simulink model "PFC_SIL_model"  (R2021a)
settings: Solver=VariableStepAuto  StartTime=0.0  StopTime=1  MaxStep=1e-5  RelTol=1e-3
values from neighbouring files (symbols this model uses):
  ki_current = 140/3    (= 46.6666666667)    [PFC_drscrete.m]
  ki_volt = 0.4    [PFC_drscrete.m]
  kp_curr = 0.027    [PFC_drscrete.m]
  kp_volt = 0.03    [PFC_drscrete.m]
  Po = 15000/3    (= 5000)    [PFC_drscrete.m]
  Ramp = 0.008    [PFC_drscrete.m]
  ramp_initial = 0.2    [PFC_drscrete.m]
  ramp_sat_max = 0.95    [PFC_drscrete.m]
  ramp_sat_min = 0.2    [PFC_drscrete.m]
  Ro = 100e3    (= 100000)    [PFC_drscrete.m]
  Softstart_th = 30    [PFC_drscrete.m]
  Vm = 400    [PFC_drscrete.m]
  Vo = 100    [PFC_drscrete.m]
undefined symbols (not defined in the file or in its folder): DiscIntNeverNeededParam, T_Finished, T_step
libraries: spsSeriesRLCBranchLib x34, simulink x19, spsMosfetLib x8, spsPWMGeneratorDCDCLib x8, spsControlledVoltageSourceLib x6, spsGroundLib x6, spsVoltageMeasurementLib x6, spsCurrentMeasurementLib x3, pid_lib x2, spsDiodeLib x2, spspowerguiLib x1
(part 1 of 2)
settings Model: Creator=houma  LastModifiedBy=prizm
settings SolverCC: AlgebraicLoopSolver=TrustRegion
settings DataIOCC: ReturnWorkspaceOutputs=off
settings DebuggingCC: SFMachineParentedDataDiag=warning  ArithmeticOperatorsInVariantConditions=warning
settings SFSimCC: SimUseLocalCustomCode=off  CustomCodeUndefinedFunction=UseInterfaceOnly
settings RTWCC: RTWUseLocalCustomCode=off

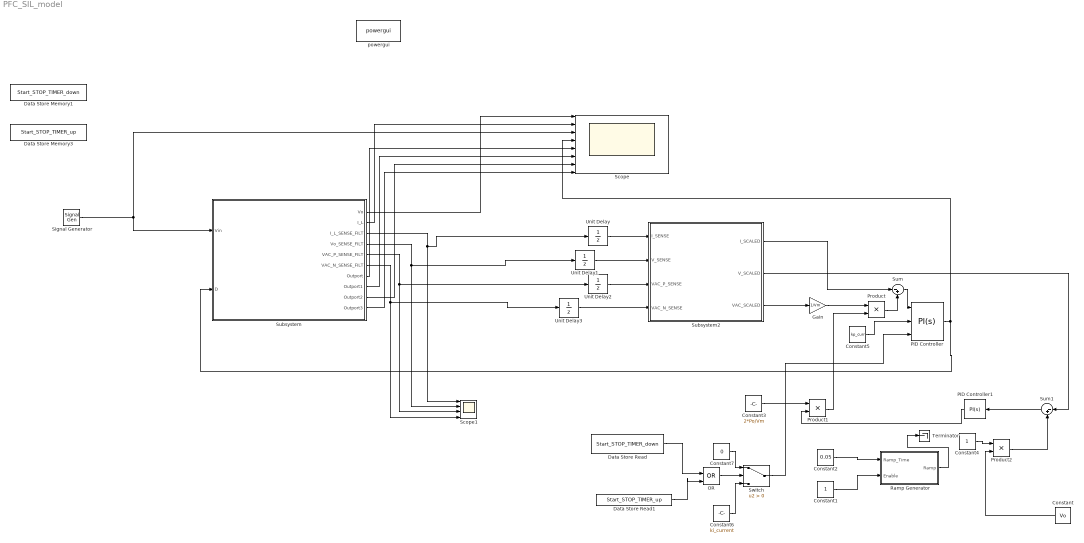
== system PFC_SIL_model ==
  Constant : Constant  Value=Vo
  Constant1 : Constant
  Constant2 : Constant  Value=0.05
  Constant3 : Constant  Value=2*Po/Vm
  Constant4 : Constant
  Constant5 : Constant  Value=kp_curr
  Constant6 : Constant  Value=ki_current
  Constant7 : Constant  Value=0
  Data Store Memory1 : DataStoreMemory  DataStoreName=Start_STOP_TIMER_down  ReadBeforeWriteMsg=warning  WriteAfterWriteMsg=warning  WriteAfterReadMsg=warning  ShowAdditionalParam=off
  Data Store Memory3 : DataStoreMemory  DataStoreName=Start_STOP_TIMER_up  ReadBeforeWriteMsg=warning  WriteAfterWriteMsg=warning  WriteAfterReadMsg=warning  ShowAdditionalParam=off
  Data Store Read : DataStoreRead  DataStoreName=Start_STOP_TIMER_down  IndexOptions=Index vector (dialog)  Indices=1  OutputSizes=1
  Data Store Read1 : DataStoreRead  DataStoreName=Start_STOP_TIMER_up  IndexOptions=Index vector (dialog)  Indices=1  OutputSizes=1
  Gain : Gain  Gain=1/Vm
  OR : Logic  Operator=OR  IconShape=distinctive  AllPortsSameDT=off  OutDataTypeStr=boolean
  PID Controller : pid_lib/PID Controller  Controller=PI  Form=Parallel  TimeDomain=Continuous-time  UseExternalTs=off  SampleTime=-1  IntegratorMethod=Forward Euler  FilterMethod=Forward Euler  ControllerParametersSource=external  P=0.027  I=140*2  D=0.0002  UseFilter=on  N=100  TunerSelectOption=Transfer Function Based (PID Tuner App)  InitialConditionSource=internal  InitialConditionForIntegrator=0  InitialConditionForFilter=0  DifferentiatorICPrevScaledInput=0  ExternalReset=none  TrackingMode=off  Kt=1  LimitOutput=on  SatLimitsSource=internal  UpperSaturationLimit=0.95  LowerSaturationLimit=0.05  LinearizeAsGain=off  AntiWindupMode=none  Kb=1  POutMin=[]  POutMax=[]  IOutMin=[]  IOutMax=[]  DOutMin=[]  DOutMax=[]  NOutMin=[]  NOutMax=[]  SumOutMin=[]  SumOutMax=[]  SaturationOutMin=[]  SaturationOutMax=[]  PParamMin=[]  PParamMax=[]  IParamMin=[]  IParamMax=[]  DParamMin=[]  DParamMax=[]  NParamMin=[]  NParamMax=[]  KbParamMin=[]  KbParamMax=[]  KtParamMin=[]  KtParamMax=[]  KbOutMin=[]  KbOutMax=[]  KtOutMin=[]  KtOutMax=[]  IntegratorOutMin=[]  IntegratorOutMax=[]  FilterOutMin=[]  FilterOutMax=[]  SumI1OutMin=[]  SumI1OutMax=[]  SumI2OutMin=[]  SumI2OutMax=[]  SumI3OutMin=[]  SumI3OutMax=[]  SumI4OutMin=[]  SumI4OutMax=[]  SumDOutMin=[]  SumDOutMax=[]  DifferentiatorOutMin=[]  DifferentiatorOutMax=[]  FilterDiffOutCoefMin=[]  FilterDiffOutCoefMax=[]  ReciprocalOutMin=[]  ReciprocalOutMax=[]  SumDenOutMin=[]  SumDenOutMax=[]  SumNumOutMin=[]  SumNumOutMax=[]  DivideOutMin=[]  DivideOutMax=[]  UdiffTsProdOutMin=[]  UdiffTsProdOutMax=[]  NTsProdOutMin=[]  NTsProdOutMax=[]  UintegralTsProdOutMin=[]  UintegralTsProdOutMax=[]  UngainTsProdOutMin=[]  UngainTsProdOutMax=[]  IntegratorContinuousStateAttributes=''  IntegratorStateMustResolveToSignalObject=off  IntegratorRTWStateStorageClass=Auto  FilterContinuousStateAttributes=''  FilterStateMustResolveToSignalObject=off  FilterRTWStateStorageClass=Auto  ParallelPVariant=ExternalParameters  IdealPVariant=Disabled  IVariant=ExternalParameters  DVariant=Disabled  IntegratorVariant=Continuous  SatVariant=Enabled  AWVariant=Passthrough  PCopyVariant=Disabled  TRVariant=Disabled  FdbkBlocksVariant=Forward  IdealPFdbkVariant=Disabled  SatFdbkVariant=Disabled  DerivativeFilterVariant=Disabled  NVariant=Disabled  NCopyVariant=Disabled_SignalSpec  FilterICVariant=Disabled  IntegratorICVariant=InternalICs  ExternalResetVariant=Disabled  TRSumVariant=Passthrough  SumFdbkVariant=Disabled  SumVariant=Sum_PI  TsampFilterVariant=InternalTs  TsampNgainVariant=Passthrough  TsampIntegralVariant=Passthrough  ExternalSaturationOutDataTypeStr=Inherit: Same as second input
  PID Controller1 : pid_lib/PID Controller  Controller=PI  Form=Parallel  TimeDomain=Continuous-time  UseExternalTs=off  SampleTime=-1  IntegratorMethod=Forward Euler  FilterMethod=Forward Euler  ControllerParametersSource=internal  P=kp_volt  I=ki_volt  D=0  UseFilter=on  N=100  TunerSelectOption=Transfer Function Based (PID Tuner App)  InitialConditionSource=internal  InitialConditionForIntegrator=0  InitialConditionForFilter=0  DifferentiatorICPrevScaledInput=0  ExternalReset=none  TrackingMode=off  Kt=1  LimitOutput=on  SatLimitsSource=internal  UpperSaturationLimit=1  LowerSaturationLimit=0  LinearizeAsGain=off  AntiWindupMode=none  Kb=1  POutMin=[]  POutMax=[]  IOutMin=[]  IOutMax=[]  DOutMin=[]  DOutMax=[]  NOutMin=[]  NOutMax=[]  SumOutMin=[]  SumOutMax=[]  SaturationOutMin=[]  SaturationOutMax=[]  PParamMin=[]  PParamMax=[]  IParamMin=[]  IParamMax=[]  DParamMin=[]  DParamMax=[]  NParamMin=[]  NParamMax=[]  KbParamMin=[]  KbParamMax=[]  KtParamMin=[]  KtParamMax=[]  KbOutMin=[]  KbOutMax=[]  KtOutMin=[]  KtOutMax=[]  IntegratorOutMin=[]  IntegratorOutMax=[]  FilterOutMin=[]  FilterOutMax=[]  SumI1OutMin=[]  SumI1OutMax=[]  SumI2OutMin=[]  SumI2OutMax=[]  SumI3OutMin=[]  SumI3OutMax=[]  SumI4OutMin=[]  SumI4OutMax=[]  SumDOutMin=[]  SumDOutMax=[]  DifferentiatorOutMin=[]  DifferentiatorOutMax=[]  FilterDiffOutCoefMin=[]  FilterDiffOutCoefMax=[]  ReciprocalOutMin=[]  ReciprocalOutMax=[]  SumDenOutMin=[]  SumDenOutMax=[]  SumNumOutMin=[]  SumNumOutMax=[]  DivideOutMin=[]  DivideOutMax=[]  UdiffTsProdOutMin=[]  UdiffTsProdOutMax=[]  NTsProdOutMin=[]  NTsProdOutMax=[]  UintegralTsProdOutMin=[]  UintegralTsProdOutMax=[]  UngainTsProdOutMin=[]  UngainTsProdOutMax=[]  IntegratorContinuousStateAttributes=''  IntegratorStateMustResolveToSignalObject=off  IntegratorRTWStateStorageClass=Auto  FilterContinuousStateAttributes=''  FilterStateMustResolveToSignalObject=off  FilterRTWStateStorageClass=Auto  ParallelPVariant=InternalParameters  IdealPVariant=Disabled  IVariant=InternalParameters  DVariant=Disabled  IntegratorVariant=Continuous  SatVariant=Enabled  AWVariant=Passthrough  PCopyVariant=Disabled  TRVariant=Disabled  FdbkBlocksVariant=Forward  IdealPFdbkVariant=Disabled  SatFdbkVariant=Disabled  DerivativeFilterVariant=Disabled  NVariant=Disabled  NCopyVariant=Disabled_SignalSpec  FilterICVariant=Disabled  IntegratorICVariant=InternalICs  ExternalResetVariant=Disabled  TRSumVariant=Passthrough  SumFdbkVariant=Disabled  SumVariant=Sum_PI  TsampFilterVariant=InternalTs  TsampNgainVariant=Passthrough  TsampIntegralVariant=Passthrough  ExternalSaturationOutDataTypeStr=Inherit: Same as second input
  Product : Product
  Product1 : Product
  Product2 : Product
  Ramp Generator : Subsystem
  Scope : Scope  NumInputPorts=8
  Scope1 : Scope  NumInputPorts=4
  Signal Generator : SignalGenerator  Amplitude=Vm  Frequency=60
  Subsystem : Subsystem
  Subsystem2 : Subsystem
  Sum : Sum  Inputs=|-+
  Sum1 : Sum  Inputs=|-+
  Switch : Switch  Criteria=u2 > Threshold
  Terminator : Terminator
  Unit Delay{,1..3} (4 alike) : UnitDelay  SampleTime=-1  HasFrameUpgradeWarning=on
  powergui : spspowerguiLib/powergui  Priority=1  SimulationMode=Continuous  SampleTime=50e-6  frequency=60  Iterations=50  frequencyindice=0  Pbase=100e6  ErrMax=1e-4  UnitsV=kV  UnitsW=MW  buscounter=0  FunctionMessages=off  echomessages=off  EnableUseOfTLC=off  CurrentSourceSwitches=off  DisableSnubberDevices=off  DisableRonSwitches=off  DisableVfSwitches=off  DisplayEquations=off  AutomaticDiscreteSolvers=off  SolverType=Tustin/Backward Euler (TBE)  Interpol=off  ExternalGateDelay=off  methode=off  Ts=100  x0status=blocks  SPID=on  SwTol=0  HookPort=off  NonlinearTolerance=1e-4  nMaxIteration=100  ContinueOnMaxIteration=off  RestoreLinks=warning  ResistiveCurrentMeasurement=off  Frange=[0:2:500]  Ylog=off  Xlog=on  ShowGrid=off  save=off  variable=ZData  structure=0  ZoomFFT=off  StartTime=0.0  cycles=1  DisplayStyle=1  fundamental=60  FreqAxis=off  MaxFrequency=1000  frequencyindicesteady=1  RmsSteady=1  display=off
  wires:
  Subsystem2/1(I_SCALED) -> Sum/1
  Subsystem/3(I_L_SENSE_FILT) -> Scope1/1, Unit Delay/1
  Gain/1 -> Product/1
  Product/1 -> Sum/2
  Subsystem/6(VAC_N_SENSE_FILT) -> Scope1/4, Unit Delay3/1
  Subsystem/4(Vo_SENSE_FILT) -> Scope1/2, Unit Delay1/1
  Subsystem2/3(VAC_SCALED) -> Gain/1
  Unit Delay/1 -> Subsystem2/1(I_SENSE)
  Unit Delay1/1 -> Subsystem2/2(V_SENSE)
  Unit Delay2/1 -> Subsystem2/3(VAC_P_SENSE)
  Subsystem/1(Vo) -> Scope/1
  Subsystem/5(VAC_P_SENSE_FILT) -> Scope1/3, Unit Delay2/1
  Unit Delay3/1 -> Subsystem2/4(VAC_N_SENSE)
  Subsystem/2(I_L) -> Scope/2
  Sum/1 -> PID Controller/1
  Signal Generator/1 -> Scope/3, Subsystem/1(Vin)
  PID Controller/1 -> Scope/4, Subsystem/2(D)
  Constant3/1 -> Product1/1
  Product1/1 -> Product/2
  Subsystem2/2(V_SCALED) -> Sum1/1
  Sum1/1 -> PID Controller1/1
  PID Controller1/1 -> Product1/2
  Constant/1 -> Product2/2
  Subsystem/7(Outport) -> Scope/5
  Subsystem/8(Outport1) -> Scope/6
  Subsystem/9(Outport2) -> Scope/7
  Subsystem/10(Outport3) -> Scope/8
  Ramp Generator/1(Ramp) -> Terminator/1
  Product2/1 -> Sum1/2
  Constant1/1 -> Ramp Generator/2(Enable)
  Constant2/1 -> Ramp Generator/1(Ramp_Time)
  Constant4/1 -> Product2/1
  Constant5/1 -> PID Controller/2
  Switch/1 -> PID Controller/3
  Data Store Read/1 -> OR/1
  Data Store Read1/1 -> OR/2
  OR/1 -> Switch/2
  Constant7/1 -> Switch/1
  Constant6/1 -> Switch/3

== system PFC_SIL_model/Ramp Generator ==
  Ramp_Time : Inport
  Enable : Inport  Port=2
  Divide : Product  Inputs=*/  RndMeth=Simplest  OutDataTypeStr=Inherit: Same as first input
  NOT : Logic  Operator=NOT  IconShape=distinctive  AllPortsSameDT=off  OutDataTypeStr=boolean
  One : Constant  SampleTime=-1
  Ramp Generator : DiscreteIntegrator  IntegratorMethod=Accumulation: Forward Euler  gainval=1  ExternalReset=sampled level  SampleTime=-1  RndMeth=Simplest  LimitOutput=on  UpperSaturationLimit=1  LowerSaturationLimit=0  ICPrevOutput=DiscIntNeverNeededParam  ICPrevScaledInput=DiscIntNeverNeededParam
  Sample_Time : Gain  Gain=0.00001  RndMeth=Simplest  OutDataTypeStr=Inherit: Same as input
  Ramp : Outport
  wires:
  Divide/1 -> Sample_Time/1
  Ramp Generator/1 -> Ramp/1  "Eps"
  Sample_Time/1 -> Ramp Generator/1
  One/1 -> Divide/1
  Ramp_Time/1 -> Divide/2
  Enable/1 -> NOT/1
  NOT/1 -> Ramp Generator/2

== system PFC_SIL_model/Subsystem ==
  Vin : Inport
  D : Inport  Port=2
  Subsystem3 : Subsystem
  Subsystem4 : Subsystem
  Subsystem5 : Subsystem
  Vo : Outport  VectorParamsAs1DForOutWhenUnconnected=off
  I_L : Outport  Port=2  VectorParamsAs1DForOutWhenUnconnected=off
  I_L_SENSE_FILT : Outport  Port=3  VectorParamsAs1DForOutWhenUnconnected=off
  Vo_SENSE_FILT : Outport  Port=4  VectorParamsAs1DForOutWhenUnconnected=off
  VAC_P_SENSE_FILT : Outport  Port=5  VectorParamsAs1DForOutWhenUnconnected=off
  VAC_N_SENSE_FILT : Outport  Port=6  VectorParamsAs1DForOutWhenUnconnected=off
  Outport : Outport  Port=7
  Outport1 : Outport  Port=8
  Outport2 : Outport  Port=9
  Outport3 : Outport  Port=10
  wires:
  Subsystem3/1(VAC_N_Sense_FILT) -> VAC_N_SENSE_FILT/1  "VAC_N_SENSE_FILT"
  Subsystem5/3(I_L_Sense_FILT) -> I_L_SENSE_FILT/1  "I_L_SENSE_FILT"
  Subsystem5/1(Vo) -> Vo/1  "Vo"
  Vin/1 -> Subsystem3/1(VAC_IN), Subsystem4/1(VAC_IN), Subsystem5/1(Vin)
  Subsystem5/4(Vo_Sense_FILT) -> Vo_SENSE_FILT/1  "Vo_SENSE_FILT"
  D/1 -> Subsystem5/2(D)
  Subsystem4/1(VAC_P_Sense_FILT) -> VAC_P_SENSE_FILT/1  "VAC_P_SENSE_FILT"
  Subsystem5/2(I_L) -> I_L/1
  Subsystem5/5(Outport) -> Outport/1
  Subsystem5/6(Outport1) -> Outport1/1
  Subsystem5/7(Outport2) -> Outport2/1
  Subsystem5/8(Outport3) -> Outport3/1

== system PFC_SIL_model/Subsystem2 ==
  I_SENSE : Inport
  V_SENSE : Inport  Port=2
  VAC_P_SENSE : Inport  Port=3
  VAC_N_SENSE : Inport  Port=4
  Gain : Gain  Gain=307.39
  Gain1 : Gain  Gain=230.79
  Gain2 : Gain  Gain=230.79
  Subsystem1 : Subsystem  mask{Gain=0.025, Vref=2.5}
      mask prompts: Gain "Gain (mV/A)"; Vref "reference Voltage"
  Sum : Sum  Inputs=|+-
  I_SCALED : Outport  VectorParamsAs1DForOutWhenUnconnected=off
  V_SCALED : Outport  Port=2  VectorParamsAs1DForOutWhenUnconnected=off
  VAC_SCALED : Outport  Port=3  VectorParamsAs1DForOutWhenUnconnected=off
  wires:
  Sum/1 -> VAC_SCALED/1  "VAC_SCALED"
  V_SENSE/1 -> Gain/1
  Subsystem1/1(I_Scaled) -> I_SCALED/1  "I_SCALED"
  Gain/1 -> V_SCALED/1  "V_SCALED"
  VAC_N_SENSE/1 -> Gain2/1
  Gain1/1 -> Sum/1
  Gain2/1 -> Sum/2
  I_SENSE/1 -> Subsystem1/1(I_ADC)
  VAC_P_SENSE/1 -> Gain1/1

== system PFC_SIL_model/Subsystem/Subsystem3 ==
  VAC_IN : Inport
  Controlled Voltage Source3 : spsControlledVoltageSourceLib/Controlled Voltage Source  Initialize=on  Source_Type=AC  Amplitude=0  Phase=0  Frequency=0  Measurements=None
  Diode1 : spsDiodeLib/Diode  Ron=0.001  Lon=0  Vf=0.8  IC=0  UseSnubber=0  Rs=1e9  Cs=0  Measurements=off
  Ground3 : spsGroundLib/Ground  LConnTagsString=a
  Series RLC Branch21 : spsSeriesRLCBranchLib/Series RLC Branch  LConnTagsString=__new0  RConnTagsString=__new0  BranchType=R  Resistance=15000  Inductance=1e-3  SetiL0=off  InitialCurrent=0  Capacitance=1e-6  Setx0=off  InitialVoltage=0  Measurements=None
  Series RLC Branch22 : spsSeriesRLCBranchLib/Series RLC Branch  LConnTagsString=__new0  RConnTagsString=__new0  BranchType=C  Resistance=4700  Inductance=1e-3  SetiL0=off  InitialCurrent=0  Capacitance=1e-9  Setx0=off  InitialVoltage=0  Measurements=None
  Series RLC Branch23 : spsSeriesRLCBranchLib/Series RLC Branch  LConnTagsString=__new0  RConnTagsString=__new0  BranchType=R  Resistance=15000  Inductance=1e-3  SetiL0=off  InitialCurrent=0  Capacitance=1e-6  Setx0=off  InitialVoltage=0  Measurements=None
  Series RLC Branch24 : spsSeriesRLCBranchLib/Series RLC Branch  LConnTagsString=__new0  RConnTagsString=__new0  BranchType=C  Resistance=4700  Inductance=1e-3  SetiL0=off  InitialCurrent=0  Capacitance=1e-9  Setx0=off  InitialVoltage=0  Measurements=None
  Series RLC Branch25 : spsSeriesRLCBranchLib/Series RLC Branch  LConnTagsString=__new0  RConnTagsString=__new0  BranchType=R  Resistance=1.08e6  Inductance=1e-3  SetiL0=off  InitialCurrent=0  Capacitance=1e-6  Setx0=off  InitialVoltage=0  Measurements=None
  Series RLC Branch26 : spsSeriesRLCBranchLib/Series RLC Branch  LConnTagsString=__new0  RConnTagsString=__new0  BranchType=R  Resistance=4700  Inductance=1e-3  SetiL0=off  InitialCurrent=0  Capacitance=1e-6  Setx0=off  InitialVoltage=0  Measurements=None
  Series RLC Branch27 : spsSeriesRLCBranchLib/Series RLC Branch  LConnTagsString=__new0  RConnTagsString=__new0  BranchType=C  Resistance=4700  Inductance=1e-3  SetiL0=off  InitialCurrent=0  Capacitance=470e-12  Setx0=off  InitialVoltage=0  Measurements=None
  Voltage Measurement3 : spsVoltageMeasurementLib/Voltage Measurement  PhasorSimulation=off  OutputType=Complex  PSBequivalent=0
  VAC_N_Sense_FILT : Outport  VectorParamsAs1DForOutWhenUnconnected=off
  wires:
  VAC_IN/1 -> Controlled Voltage Source3/1
  Voltage Measurement3/1 -> VAC_N_Sense_FILT/1  "VAC_N_Sense_FILT"
  connections:
  Diode1/RConn1 -- Series RLC Branch25/LConn1
  Series RLC Branch26/RConn1 -- Series RLC Branch27/RConn1 -- Series RLC Branch22/RConn1 -- Series RLC Branch24/RConn1 -- Voltage Measurement3/LConn2 -- Ground3/LConn1 -- Controlled Voltage Source3/RConn1
  Controlled Voltage Source3/LConn1 -- Diode1/LConn1
  Series RLC Branch23/RConn1 -- Voltage Measurement3/LConn1 -- Series RLC Branch24/LConn1
  Series RLC Branch25/RConn1 -- Series RLC Branch27/LConn1 -- Series RLC Branch21/LConn1 -- Series RLC Branch26/LConn1
  Series RLC Branch21/RConn1 -- Series RLC Branch22/LConn1 -- Series RLC Branch23/LConn1

== system PFC_SIL_model/Subsystem/Subsystem4 ==
  VAC_IN : Inport
  Controlled Voltage Source2 : spsControlledVoltageSourceLib/Controlled Voltage Source  Initialize=on  Source_Type=AC  Amplitude=0  Phase=0  Frequency=0  Measurements=None
  Current Measurement : spsCurrentMeasurementLib/Current Measurement  PhasorSimulation=off  OutputType=Complex  PSBequivalent=0
  Diode : spsDiodeLib/Diode  Ron=0.001  Lon=0  Vf=0.8  IC=0  UseSnubber=0  Rs=1e9  Cs=0  Measurements=off
  Ground2 : spsGroundLib/Ground  LConnTagsString=a
  Scope : Scope
  Series RLC Branch14 : spsSeriesRLCBranchLib/Series RLC Branch  LConnTagsString=__new0  RConnTagsString=__new0  BranchType=R  Resistance=15000  Inductance=1e-3  SetiL0=off  InitialCurrent=0  Capacitance=1e-6  Setx0=off  InitialVoltage=0  Measurements=None
  Series RLC Branch15 : spsSeriesRLCBranchLib/Series RLC Branch  LConnTagsString=__new0  RConnTagsString=__new0  BranchType=C  Resistance=4700  Inductance=1e-3  SetiL0=off  InitialCurrent=0  Capacitance=1e-9  Setx0=off  InitialVoltage=0  Measurements=None
  Series RLC Branch16 : spsSeriesRLCBranchLib/Series RLC Branch  LConnTagsString=__new0  RConnTagsString=__new0  BranchType=R  Resistance=15000  Inductance=1e-3  SetiL0=off  InitialCurrent=0  Capacitance=1e-6  Setx0=off  InitialVoltage=0  Measurements=None
  Series RLC Branch17 : spsSeriesRLCBranchLib/Series RLC Branch  LConnTagsString=__new0  RConnTagsString=__new0  BranchType=C  Resistance=4700  Inductance=1e-3  SetiL0=off  InitialCurrent=0  Capacitance=1e-9  Setx0=off  InitialVoltage=0  Measurements=None
  Series RLC Branch18 : spsSeriesRLCBranchLib/Series RLC Branch  LConnTagsString=__new0  RConnTagsString=__new0  BranchType=R  Resistance=1.08e6  Inductance=1e-3  SetiL0=off  InitialCurrent=0  Capacitance=1e-6  Setx0=off  InitialVoltage=0  Measurements=None
  Series RLC Branch19 : spsSeriesRLCBranchLib/Series RLC Branch  LConnTagsString=__new0  RConnTagsString=__new0  BranchType=R  Resistance=4700  Inductance=1e-3  SetiL0=off  InitialCurrent=0  Capacitance=1e-6  Setx0=off  InitialVoltage=0  Measurements=None
  Series RLC Branch20 : spsSeriesRLCBranchLib/Series RLC Branch  LConnTagsString=__new0  RConnTagsString=__new0  BranchType=C  Resistance=4700  Inductance=1e-3  SetiL0=off  InitialCurrent=0  Capacitance=470e-12  Setx0=off  InitialVoltage=0  Measurements=None
  Voltage Measurement2 : spsVoltageMeasurementLib/Voltage Measurement  PhasorSimulation=off  OutputType=Complex  PSBequivalent=0
  VAC_P_Sense_FILT : Outport  VectorParamsAs1DForOutWhenUnconnected=off
  wires:
  VAC_IN/1 -> Controlled Voltage Source2/1
  Voltage Measurement2/1 -> VAC_P_Sense_FILT/1  "VAC_P_Sense_FILT"
  Current Measurement/1 -> Scope/1
  connections:
  Current Measurement/LConn1 -- Series RLC Branch18/RConn1
  Series RLC Branch19/LConn1 -- Series RLC Branch20/LConn1 -- Series RLC Branch14/LConn1 -- Current Measurement/RConn1
  Series RLC Branch14/RConn1 -- Series RLC Branch15/LConn1 -- Series RLC Branch16/LConn1
  Series RLC Branch16/RConn1 -- Voltage Measurement2/LConn1 -- Series RLC Branch17/LConn1
  Ground2/LConn1 -- Series RLC Branch20/RConn1 -- Series RLC Branch15/RConn1 -- Series RLC Branch17/RConn1 -- Voltage Measurement2/LConn2 -- Series RLC Branch19/RConn1 -- Controlled Voltage Source2/LConn1
  Series RLC Branch18/LConn1 -- Diode/RConn1
  Diode/LConn1 -- Controlled Voltage Source2/RConn1

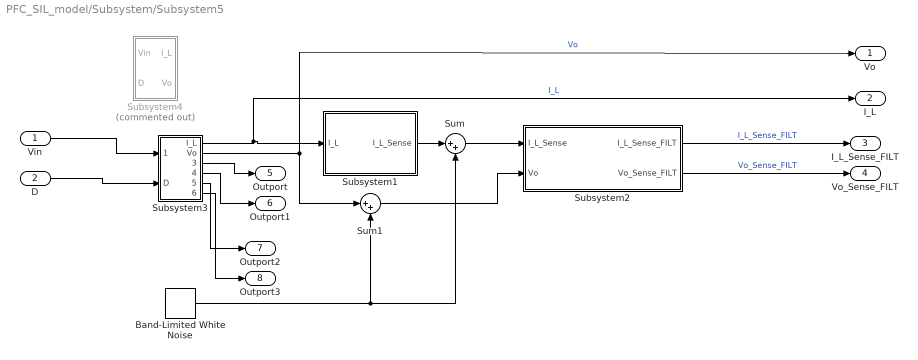
== system PFC_SIL_model/Subsystem/Subsystem5 ==
  Vin : Inport
  D : Inport  Port=2
  Band-Limited White Noise : simulink/Sources/Band-Limited White Noise  Cov=[0]  Ts=1/100e3  seed=[23341]
  Subsystem1 : Subsystem  mask{G_current=0.025, Vref=2.5}
      mask prompts: G_current "Current Gain (V/A)"; Vref "Reference Voltage"
  Subsystem2 : Subsystem
  Subsystem3 : Subsystem  mask{Lo=450e-6, Co=1.1e-3}
      mask prompts: Lo "PFC Inductance"; Co "Bus Capacitance"
  Subsystem4 : Subsystem  Commented=on  mask{Lo=450e-6, Co=1.1e-3}
      mask prompts: Lo "PFC Inductance"; Co "Bus Capacitance"
  Sum : Sum  Inputs=|++
  Sum1 : Sum  Inputs=|++
  Vo : Outport  VectorParamsAs1DForOutWhenUnconnected=off
  I_L : Outport  Port=2  VectorParamsAs1DForOutWhenUnconnected=off
  I_L_Sense_FILT : Outport  Port=3  VectorParamsAs1DForOutWhenUnconnected=off
  Vo_Sense_FILT : Outport  Port=4  VectorParamsAs1DForOutWhenUnconnected=off
  Outport : Outport  Port=5
  Outport1 : Outport  Port=6
  Outport2 : Outport  Port=7
  Outport3 : Outport  Port=8
  wires:
  D/1 -> Subsystem3/2(D)
  Subsystem2/2(Vo_Sense_FILT) -> Vo_Sense_FILT/1  "Vo_Sense_FILT"
  Subsystem2/1(I_L_Sense_FILT) -> I_L_Sense_FILT/1  "I_L_Sense_FILT"
  Vin/1 -> Subsystem3/1(Vin)
  Subsystem3/2(Vo) -> Sum1/1, Vo/1  "Vo"
  Subsystem3/1(I_L) -> I_L/1, Subsystem1/1(I_L)  "I_L"
  Band-Limited White Noise/1 -> Sum1/2, Sum/2
  Subsystem1/1(I_L_Sense) -> Sum/1
  Sum/1 -> Subsystem2/1(I_L_Sense)
  Sum1/1 -> Subsystem2/2(Vo)
  Subsystem3/3(Outport) -> Outport/1
  Subsystem3/4(Outport1) -> Outport1/1
  Subsystem3/5(Outport2) -> Outport2/1
  Subsystem3/6(Outport3) -> Outport3/1

== system PFC_SIL_model/Subsystem2/Subsystem1 ==
  I_ADC : Inport
  Constant3 : Constant  Value=Vref
  Gain : Gain  Gain=2
  Gain1 : Gain  Gain=1/Gain
  Sum : Sum  Inputs=|+-
  I_Scaled : Outport  VectorParamsAs1DForOutWhenUnconnected=off
  wires:
  Gain/1 -> Sum/1
  Constant3/1 -> Sum/2
  Gain1/1 -> I_Scaled/1  "I_Scaled"
  Sum/1 -> Gain1/1
  I_ADC/1 -> Gain/1

== system PFC_SIL_model/Subsystem/Subsystem5/Subsystem1 ==
  I_L : Inport
  Constant : Constant  Value=Vref
  Gain : Gain  Gain=G_current
  Sum : Sum  Inputs=|++
  I_L_Sense : Outport  VectorParamsAs1DForOutWhenUnconnected=off
  wires:
  Sum/1 -> I_L_Sense/1  "I_L_Sense"
  I_L/1 -> Gain/1
  Gain/1 -> Sum/1
  Constant/1 -> Sum/2

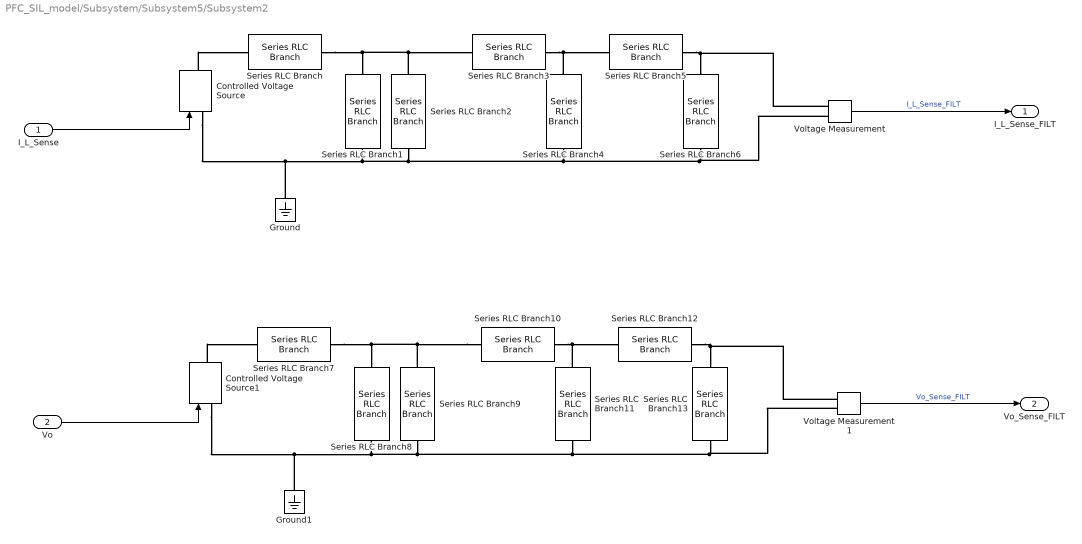
== system PFC_SIL_model/Subsystem/Subsystem5/Subsystem2 ==
  I_L_Sense : Inport
  Vo : Inport  Port=2
  Controlled Voltage Source : spsControlledVoltageSourceLib/Controlled Voltage Source  Initialize=on  Source_Type=AC  Amplitude=0  Phase=0  Frequency=0  Measurements=None
  Controlled Voltage Source1 : spsControlledVoltageSourceLib/Controlled Voltage Source  Initialize=on  Source_Type=AC  Amplitude=0  Phase=0  Frequency=0  Measurements=None
  Ground : spsGroundLib/Ground  LConnTagsString=a
  Ground1 : spsGroundLib/Ground  LConnTagsString=a
  Series RLC Branch{,1,3,5,8,10,12} (7 alike) : spsSeriesRLCBranchLib/Series RLC Branch  LConnTagsString=__new0  RConnTagsString=__new0  BranchType=R  Resistance=4700  Inductance=1e-3  SetiL0=off  InitialCurrent=0  Capacitance=1e-6  Setx0=off  InitialVoltage=0  Measurements=None
  Series RLC Branch{4,6,11,13} (4 alike) : spsSeriesRLCBranchLib/Series RLC Branch  LConnTagsString=__new0  RConnTagsString=__new0  BranchType=C  Resistance=4700  Inductance=1e-3  SetiL0=off  InitialCurrent=0  Capacitance=1e-9  Setx0=off  InitialVoltage=0  Measurements=None
  Series RLC Branch2 : spsSeriesRLCBranchLib/Series RLC Branch  LConnTagsString=__new0  RConnTagsString=__new0  BranchType=C  Resistance=4700  Inductance=1e-3  SetiL0=off  InitialCurrent=0  Capacitance=470e-12  Setx0=off  InitialVoltage=0  Measurements=None
  Series RLC Branch7 : spsSeriesRLCBranchLib/Series RLC Branch  LConnTagsString=__new0  RConnTagsString=__new0  BranchType=R  Resistance=1.44e6  Inductance=1e-3  SetiL0=off  InitialCurrent=0  Capacitance=1e-6  Setx0=off  InitialVoltage=0  Measurements=None
  Series RLC Branch9 : spsSeriesRLCBranchLib/Series RLC Branch  LConnTagsString=__new0  RConnTagsString=__new0  BranchType=C  Resistance=4700  Inductance=1e-3  SetiL0=off  InitialCurrent=0  Capacitance=470e-12  Setx0=off  InitialVoltage=0  Measurements=None
  Voltage Measurement : spsVoltageMeasurementLib/Voltage Measurement  PhasorSimulation=off  OutputType=Complex  PSBequivalent=0
  Voltage Measurement1 : spsVoltageMeasurementLib/Voltage Measurement  PhasorSimulation=off  OutputType=Complex  PSBequivalent=0
  I_L_Sense_FILT : Outport  VectorParamsAs1DForOutWhenUnconnected=off
  Vo_Sense_FILT : Outport  Port=2  VectorParamsAs1DForOutWhenUnconnected=off
  wires:
  I_L_Sense/1 -> Controlled Voltage Source/1
  Voltage Measurement/1 -> I_L_Sense_FILT/1  "I_L_Sense_FILT"
  Vo/1 -> Controlled Voltage Source1/1
  Voltage Measurement1/1 -> Vo_Sense_FILT/1  "Vo_Sense_FILT"
  connections:
  Series RLC Branch3/RConn1 -- Series RLC Branch4/LConn1 -- Series RLC Branch5/LConn1
  Series RLC Branch5/RConn1 -- Voltage Measurement/LConn1 -- Series RLC Branch6/LConn1
  Controlled Voltage Source/LConn1 -- Ground/LConn1 -- Voltage Measurement/LConn2 -- Series RLC Branch6/RConn1 -- Series RLC Branch4/RConn1 -- Series RLC Branch2/RConn1 -- Series RLC Branch1/RConn1
  Series RLC Branch/RConn1 -- Series RLC Branch2/LConn1 -- Series RLC Branch3/LConn1 -- Series RLC Branch1/LConn1
  Controlled Voltage Source/RConn1 -- Series RLC Branch/LConn1
  Voltage Measurement1/LConn2 -- Series RLC Branch13/RConn1 -- Series RLC Branch11/RConn1 -- Ground1/LConn1 -- Controlled Voltage Source1/LConn1 -- Series RLC Branch8/RConn1 -- Series RLC Branch9/RConn1
  Series RLC Branch10/LConn1 -- Series RLC Branch9/LConn1 -- Series RLC Branch8/LConn1 -- Series RLC Branch7/RConn1
  Series RLC Branch11/LConn1 -- Series RLC Branch12/LConn1 -- Series RLC Branch10/RConn1
  Voltage Measurement1/LConn1 -- Series RLC Branch13/LConn1 -- Series RLC Branch12/RConn1
  Controlled Voltage Source1/RConn1 -- Series RLC Branch7/LConn1

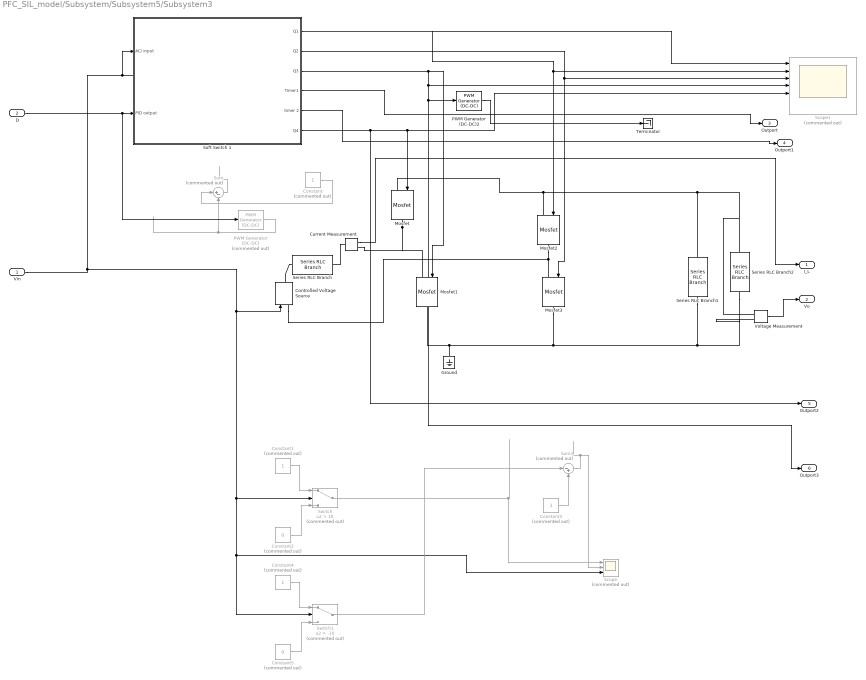
== system PFC_SIL_model/Subsystem/Subsystem5/Subsystem3 ==
  Vin : Inport
  D : Inport  Port=2
  Constant{,1,3..4} (4 alike) : Constant  Commented=on
  Constant2 : Constant  Commented=on  Value=0
  Constant5 : Constant  Commented=on  Value=0
  Controlled Voltage Source : spsControlledVoltageSourceLib/Controlled Voltage Source  Initialize=on  Source_Type=AC  Amplitude=0  Phase=0  Frequency=0  Measurements=None
  Current Measurement : spsCurrentMeasurementLib/Current Measurement  PhasorSimulation=off  OutputType=Complex  PSBequivalent=0
  Ground : spsGroundLib/Ground  LConnTagsString=a
  Mosfet{,1..3} (4 alike) : spsMosfetLib/Mosfet  Ron=0.1  Lon=0  Rd=0.01  Vfd=2  IC=0  Rs=1e5  Cs=inf  Measurements=off
  PWM Generator (DC-DC) : spsPWMGeneratorDCDCLib/PWM Generator (DC-DC)  Commented=on  Fsw=65e3  Ts=0
  PWM Generator (DC-DC)2 : spsPWMGeneratorDCDCLib/PWM Generator (DC-DC)  Fsw=65e3  Ts=0
  Scope : Scope  Commented=on  NumInputPorts=3
  Scope1 : Scope  Commented=on  NumInputPorts=7
  Series RLC Branch : spsSeriesRLCBranchLib/Series RLC Branch  LConnTagsString=__new0  RConnTagsString=__new0  BranchType=L  Resistance=1  Inductance=450e-6  SetiL0=off  InitialCurrent=0  Capacitance=1e-6  Setx0=off  InitialVoltage=0  Measurements=None
  Series RLC Branch1 : spsSeriesRLCBranchLib/Series RLC Branch  LConnTagsString=__new0  RConnTagsString=__new0  BranchType=C  Resistance=1  Inductance=450e-6  SetiL0=off  InitialCurrent=0  Capacitance=1e-3  Setx0=on  InitialVoltage=350  Measurements=None
  Series RLC Branch2 : spsSeriesRLCBranchLib/Series RLC Branch  LConnTagsString=__new0  RConnTagsString=__new0  BranchType=R  Resistance=Ro  Inductance=450e-6  SetiL0=off  InitialCurrent=0  Capacitance=1e-3  Setx0=off  InitialVoltage=0  Measurements=None
  Soft Switch 1 : Subsystem
  Sum : Sum  Commented=on  Inputs=|+-
  Sum1 : Sum  Commented=on  Inputs=|-+
  Switch : Switch  Commented=on  Criteria=u2 > Threshold  Threshold=10
  Switch1 : Switch  Commented=on  Criteria=u2 > Threshold  Threshold=-10
  Terminator : Terminator
  Voltage Measurement : spsVoltageMeasurementLib/Voltage Measurement  PhasorSimulation=off  OutputType=Complex  PSBequivalent=0
  I_L : Outport  VectorParamsAs1DForOutWhenUnconnected=off
  Vo : Outport  Port=2  VectorParamsAs1DForOutWhenUnconnected=off
  Outport : Outport  Port=3
  Outport1 : Outport  Port=4
  Outport2 : Outport  Port=5
  Outport3 : Outport  Port=6
  wires:
  Constant/1 -> Sum/1
  Sum/1 -> ?
  Current Measurement/1 -> I_L/1
  Voltage Measurement/1 -> Vo/1
  Constant1/1 -> Switch/1
  Constant2/1 -> Switch/3
  Switch/1 -> Scope/1
  Constant3/1 -> Sum1/2
  Sum1/1 -> Scope/2
  Constant5/1 -> Switch1/3
  Constant4/1 -> Switch1/1
  Vin/1 -> Controlled Voltage Source/1, Scope/3, Switch1/2, Switch/2, Scope1/1, Soft Switch 1/1(AC/ input)
  Switch1/1 -> Sum1/1
  Soft Switch 1/4(Timer1) -> Outport/1
  Soft Switch 1/3(Q3) -> Mosfet1/1, Outport3/1, PWM Generator (DC-DC)2/1, Scope1/4
  Soft Switch 1/1(Q1) -> Mosfet2/1, Scope1/2
  Soft Switch 1/2(Q2) -> Mosfet3/1, Scope1/3
  PWM Generator (DC-DC)/1 -> Sum/2
  PWM Generator (DC-DC)2/1 -> Terminator/1
  Soft Switch 1/5(timer 2) -> Outport1/1
  D/1 -> PWM Generator (DC-DC)/1, Soft Switch 1/2(PID output)
  Soft Switch 1/6(Q4) -> Outport2/1, Scope1/5, Mosfet/1
  connections:
  Controlled Voltage Source/RConn1 -- Series RLC Branch/LConn1
  Mosfet/RConn1 -- Mosfet1/LConn1 -- Current Measurement/RConn1
  Series RLC Branch1/LConn1 -- Series RLC Branch2/LConn1 -- Voltage Measurement/LConn1 -- Mosfet2/LConn1 -- Mosfet/LConn1
  Series RLC Branch1/RConn1 -- Series RLC Branch2/RConn1 -- Voltage Measurement/LConn2 -- Mosfet3/RConn1 -- Ground/LConn1 -- Mosfet1/RConn1
  Controlled Voltage Source/LConn1 -- Mosfet2/RConn1 -- Mosfet3/LConn1
  Series RLC Branch/RConn1 -- Current Measurement/LConn1

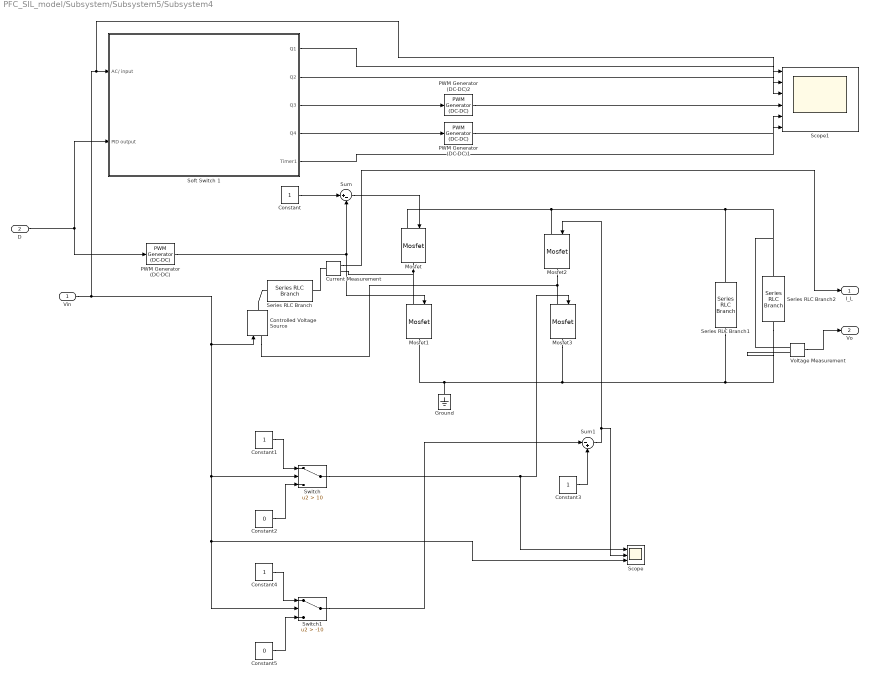
== system PFC_SIL_model/Subsystem/Subsystem5/Subsystem4 ==
  Vin : Inport
  D : Inport  Port=2
  Constant{,1,3..4} (4 alike) : Constant
  Constant2 : Constant  Value=0
  Constant5 : Constant  Value=0
  Controlled Voltage Source : spsControlledVoltageSourceLib/Controlled Voltage Source  Initialize=on  Source_Type=AC  Amplitude=0  Phase=0  Frequency=0  Measurements=None
  Current Measurement : spsCurrentMeasurementLib/Current Measurement  PhasorSimulation=off  OutputType=Complex  PSBequivalent=0
  Ground : spsGroundLib/Ground  LConnTagsString=a
  Mosfet{,1..3} (4 alike) : spsMosfetLib/Mosfet  Ron=0.1  Lon=0  Rd=0.01  Vfd=2  IC=0  Rs=1e5  Cs=inf  Measurements=off
  PWM Generator (DC-DC) : spsPWMGeneratorDCDCLib/PWM Generator (DC-DC)  Fsw=65e3  Ts=0
  PWM Generator (DC-DC)1 : spsPWMGeneratorDCDCLib/PWM Generator (DC-DC)  Fsw=65e3  Ts=0
  PWM Generator (DC-DC)2 : spsPWMGeneratorDCDCLib/PWM Generator (DC-DC)  Fsw=65e3  Ts=0
  Scope : Scope  NumInputPorts=3
  Scope1 : Scope  NumInputPorts=6
  Series RLC Branch : spsSeriesRLCBranchLib/Series RLC Branch  LConnTagsString=__new0  RConnTagsString=__new0  BranchType=L  Resistance=1  Inductance=450e-6  SetiL0=off  InitialCurrent=0  Capacitance=1e-6  Setx0=off  InitialVoltage=0  Measurements=None
  Series RLC Branch1 : spsSeriesRLCBranchLib/Series RLC Branch  LConnTagsString=__new0  RConnTagsString=__new0  BranchType=C  Resistance=1  Inductance=450e-6  SetiL0=off  InitialCurrent=0  Capacitance=1e-3  Setx0=on  InitialVoltage=350  Measurements=None
  Series RLC Branch2 : spsSeriesRLCBranchLib/Series RLC Branch  LConnTagsString=__new0  RConnTagsString=__new0  BranchType=R  Resistance=Ro  Inductance=450e-6  SetiL0=off  InitialCurrent=0  Capacitance=1e-3  Setx0=off  InitialVoltage=0  Measurements=None
  Soft Switch 1 : Subsystem
  Sum : Sum  Inputs=|+-
  Sum1 : Sum  Inputs=|-+
  Switch : Switch  Criteria=u2 > Threshold  Threshold=10
  Switch1 : Switch  Criteria=u2 > Threshold  Threshold=-10
  Voltage Measurement : spsVoltageMeasurementLib/Voltage Measurement  PhasorSimulation=off  OutputType=Complex  PSBequivalent=0
  I_L : Outport  VectorParamsAs1DForOutWhenUnconnected=off
  Vo : Outport  Port=2  VectorParamsAs1DForOutWhenUnconnected=off
  wires:
  D/1 -> PWM Generator (DC-DC)/1, Soft Switch 1/2(PID output)
  Constant/1 -> Sum/1
  Sum/1 -> Mosfet/1
  Current Measurement/1 -> I_L/1
  Voltage Measurement/1 -> Vo/1
  Constant1/1 -> Switch/1
  Constant2/1 -> Switch/3
  Switch/1 -> Mosfet3/1, Scope/1
  Constant3/1 -> Sum1/2
  Sum1/1 -> Mosfet2/1, Scope/2
  Constant5/1 -> Switch1/3
  Constant4/1 -> Switch1/1
  Vin/1 -> Scope1/1, Soft Switch 1/1(AC/ input), Scope/3, Switch1/2, Switch/2, Controlled Voltage Source/1
  Switch1/1 -> Sum1/1
  Soft Switch 1/4(Q4) -> PWM Generator (DC-DC)1/1
  Soft Switch 1/5(Timer1) -> Scope1/6
  Soft Switch 1/3(Q3) -> PWM Generator (DC-DC)2/1
  Soft Switch 1/1(Q1) -> Scope1/2
  Soft Switch 1/2(Q2) -> Scope1/3
  PWM Generator (DC-DC)/1 -> Sum/2, Mosfet1/1
  PWM Generator (DC-DC)1/1 -> Scope1/5
  PWM Generator (DC-DC)2/1 -> Scope1/4
  connections:
  Controlled Voltage Source/RConn1 -- Series RLC Branch/LConn1
  Mosfet/RConn1 -- Mosfet1/LConn1 -- Current Measurement/RConn1
  Series RLC Branch1/LConn1 -- Series RLC Branch2/LConn1 -- Voltage Measurement/LConn1 -- Mosfet2/LConn1 -- Mosfet/LConn1
  Series RLC Branch1/RConn1 -- Series RLC Branch2/RConn1 -- Voltage Measurement/LConn2 -- Mosfet3/RConn1 -- Ground/LConn1 -- Mosfet1/RConn1
  Controlled Voltage Source/LConn1 -- Mosfet2/RConn1 -- Mosfet3/LConn1
  Series RLC Branch/RConn1 -- Current Measurement/LConn1

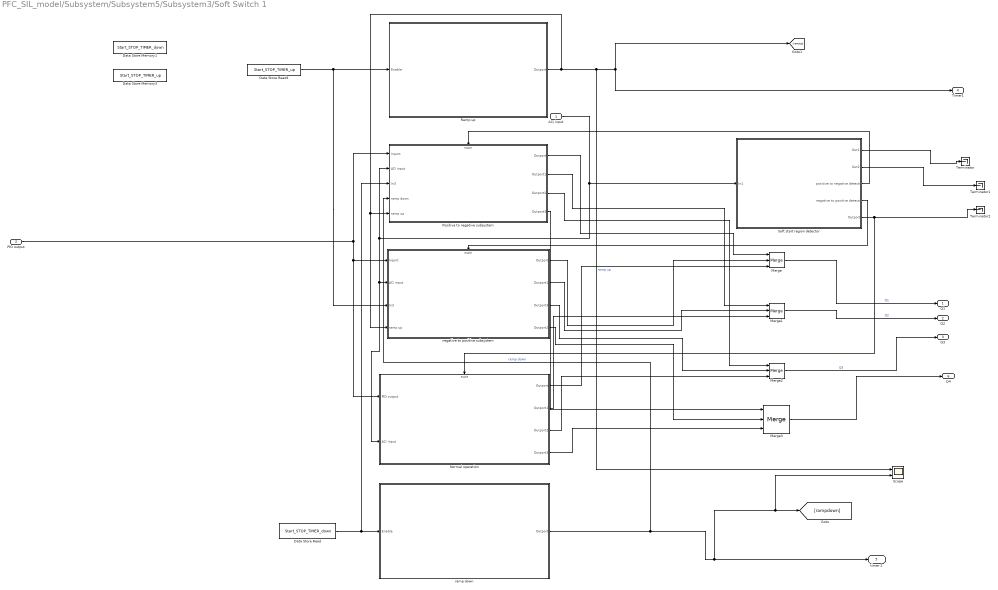
== system PFC_SIL_model/Subsystem/Subsystem5/Subsystem3/Soft Switch 1 ==
  AC/ input : Inport
  PID output : Inport  Port=2
  Data Store Memory1 : DataStoreMemory  DataStoreName=Start_STOP_TIMER_down  ReadBeforeWriteMsg=warning  WriteAfterWriteMsg=warning  WriteAfterReadMsg=warning  ShowAdditionalParam=off
  Data Store Memory3 : DataStoreMemory  DataStoreName=Start_STOP_TIMER_up  ReadBeforeWriteMsg=warning  WriteAfterWriteMsg=warning  WriteAfterReadMsg=warning  ShowAdditionalParam=off
  Data Store Read : DataStoreRead  DataStoreName=Start_STOP_TIMER_down  IndexOptions=Index vector (dialog)  Indices=1  OutputSizes=1
  Data Store Read4 : DataStoreRead  DataStoreName=Start_STOP_TIMER_up  IndexOptions=Index vector (dialog)  Indices=1  OutputSizes=1
  Merge{,1..3} (4 alike) : Merge  Inputs=3
  "Normal operation " : Subsystem  TreatAsAtomicUnit=on
  "Positive to negative subsystem " : Subsystem  TreatAsAtomicUnit=on
  "Ramp up " : Subsystem
  Scope : Scope  NumInputPorts=2
  "Soft start region detector " : Subsystem
  Terminator : Terminator
  Terminator1 : Terminator
  Terminator2 : Terminator
  "negative to positive subsystem " : Subsystem  TreatAsAtomicUnit=on
  ramp down : Subsystem
  Q1 : Outport
  Q2 : Outport  Port=2
  Q3 : Outport  Port=3
  Timer1 : Outport  Port=4
  timer 2 : Outport  Port=5
  Q4 : Outport  Port=6
  wires:
  PID output/1 -> "Positive to negative subsystem "/1(Inport), "Normal operation "/1(PID output), "negative to positive subsystem "/1(Inport)
  "Soft start region detector "/2(Out2) -> Terminator1/1
  "Soft start region detector "/4(negative to positive detector) -> "negative to positive subsystem "/Enable
  AC/ input/1 -> "Normal operation "/2(AC/ input), "negative to positive subsystem "/2(AC/ input), "Positive to negative subsystem "/2(AC/ input), "Soft start region detector "/1(In1)
  Data Store Read4/1 -> "negative to positive subsystem "/3(In3), "Ramp up "/1(Enable)
  "Soft start region detector "/1(Out1) -> Terminator/1
  Merge2/1 -> Q3/1  "Q3"
  "Soft start region detector "/3(positive to negative detector) -> "Positive to negative subsystem "/Enable
  Merge/1 -> Q1/1  "Q1"
  "Ramp up "/1(Outport) -> "Positive to negative subsystem "/5(ramp up), "negative to positive subsystem "/4("ramp up "), Scope/1, [rampup], Timer1/1  "ramp up"
  Merge1/1 -> Q2/1  "Q2"
  "Soft start region detector "/5(Outport) -> Terminator2/1, "Normal operation "/Enable
  "Positive to negative subsystem "/1(Outport) -> Merge/1
  "negative to positive subsystem "/1(Outport) -> Merge/2
  "Normal operation "/1(Outport) -> Merge/3
  "Positive to negative subsystem "/2(Outport1) -> Merge1/1
  "negative to positive subsystem "/2(Outport1) -> Merge1/2
  "Normal operation "/2(Outport1) -> Merge1/3
  "Positive to negative subsystem "/3(Outport2) -> Merge2/1
  "Normal operation "/3(Outport2) -> Merge2/3
  Data Store Read/1 -> "Positive to negative subsystem "/3(In3), ramp down/1(Enable)
  ramp down/1(Outport) -> "Positive to negative subsystem "/4("ramp down "), Scope/2, [rampdown], timer 2/1  "ramp down"
  "negative to positive subsystem "/3(Outport3) -> Merge2/2
  "Normal operation "/4(Outport3) -> Merge3/3
  "negative to positive subsystem "/4(Outport2) -> Merge3/2
  "Positive to negative subsystem "/4(Outport3) -> Merge3/1
  Merge3/1 -> Q4/1

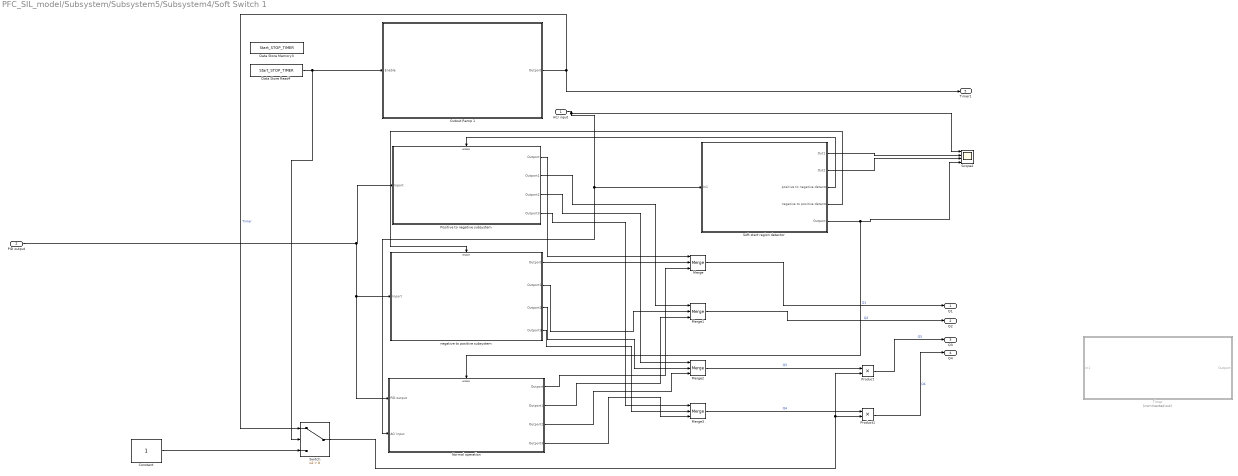
== system PFC_SIL_model/Subsystem/Subsystem5/Subsystem4/Soft Switch 1 ==
  AC/ input : Inport
  PID output : Inport  Port=2
  Constant : Constant
  Data Store Memory3 : DataStoreMemory  DataStoreName=Start_STOP_TIMER  ReadBeforeWriteMsg=warning  WriteAfterWriteMsg=warning  WriteAfterReadMsg=warning  ShowAdditionalParam=off
  Data Store Read4 : DataStoreRead  DataStoreName=Start_STOP_TIMER  IndexOptions=Index vector (dialog)  Indices=1  OutputSizes=1
  Merge{,1..3} (4 alike) : Merge  Inputs=3
  "Normal operation " : Subsystem  TreatAsAtomicUnit=on
  Outout Ramp 1 : Subsystem
  "Positive to negative subsystem " : Subsystem  TreatAsAtomicUnit=on
  Product : Product
  Product1 : Product
  Scope2 : Scope  NumInputPorts=4
  "Soft start region detector " : Subsystem
  Switch : Switch  Criteria=u2 > Threshold
  Timer : Subsystem  Commented=on
  "negative to positive subsystem " : Subsystem  TreatAsAtomicUnit=on
  Q1 : Outport
  Q2 : Outport  Port=2
  Q3 : Outport  Port=3
  Q4 : Outport  Port=4
  Timer1 : Outport  Port=5
  wires:
  PID output/1 -> "Positive to negative subsystem "/1(Inport), "Normal operation "/1(PID output), "negative to positive subsystem "/1(Inport)
  "Soft start region detector "/2(Out2) -> Scope2/3
  "Soft start region detector "/4(negative to positive detector) -> "negative to positive subsystem "/Enable
  Merge3/1 -> Product1/1  "Q4"
  AC/ input/1 -> "Normal operation "/2(AC/ input), "Soft start region detector "/1(In1), Scope2/1
  Data Store Read4/1 -> Switch/2, Outout Ramp 1/1(Enable)
  Product1/1 -> Q4/1  "Q4"
  "Soft start region detector "/1(Out1) -> Scope2/2
  Merge2/1 -> Product/1  "Q3"
  Constant/1 -> Switch/3
  "Soft start region detector "/3(positive to negative detector) -> "Positive to negative subsystem "/Enable
  Merge/1 -> Q1/1  "Q1"
  Outout Ramp 1/1(Outport) -> Switch/1, Timer1/1  "Timer"
  Merge1/1 -> Q2/1  "Q2"
  Product/1 -> Q3/1  "Q3"
  "Soft start region detector "/5(Outport) -> Scope2/4, "Normal operation "/Enable
  "Positive to negative subsystem "/1(Outport) -> Merge/1
  "negative to positive subsystem "/1(Outport) -> Merge/2
  "Normal operation "/1(Outport) -> Merge/3
  "Positive to negative subsystem "/2(Outport1) -> Merge1/1
  "negative to positive subsystem "/2(Outport1) -> Merge1/2
  "Normal operation "/2(Outport1) -> Merge1/3
  "Positive to negative subsystem "/3(Outport2) -> Merge2/1
  "Normal operation "/3(Outport2) -> Merge2/3
  "negative to positive subsystem "/3(Outport2) -> Merge2/2
  "Normal operation "/4(Outport3) -> Merge3/3
  "negative to positive subsystem "/4(Outport3) -> Merge3/2
  "Positive to negative subsystem "/4(Outport3) -> Merge3/1
  Switch/1 -> Product/2, Product1/2

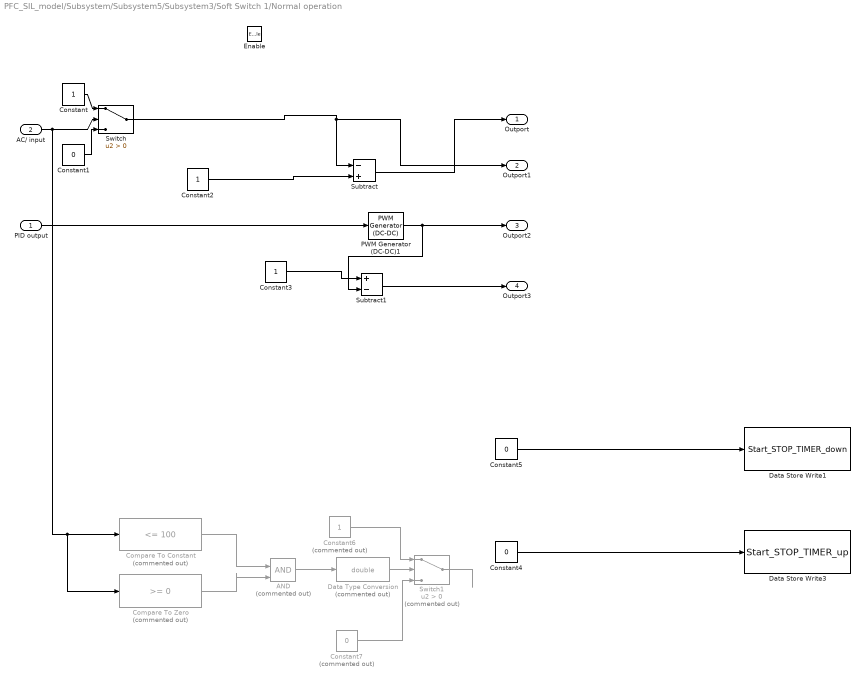
== system PFC_SIL_model/Subsystem/Subsystem5/Subsystem3/Soft Switch 1/Normal operation  ==
  PID output : Inport
  AC/ input : Inport  Port=2
  Enable : EnablePort
  AND : Logic  Commented=on  IconShape=distinctive  AllPortsSameDT=off  OutDataTypeStr=boolean
  Compare To Constant : simulink/Logic and Bit Operations/Compare To Constant  Commented=on  relop=<=  const=100  OutDataTypeStr=boolean
  Compare To Zero : simulink/Logic and Bit Operations/Compare To Zero  Commented=on  relop=>=  OutDataTypeStr=boolean
  Constant : Constant
  Constant1 : Constant  Value=0
  Constant2 : Constant
  Constant3 : Constant
  Constant4 : Constant  Value=0
  Constant5 : Constant  Value=0
  Constant6 : Constant  Commented=on
  Constant7 : Constant  Commented=on  Value=0
  Data Store Write1 : DataStoreWrite  DataStoreName=Start_STOP_TIMER_down  IndexOptions=Index vector (dialog)  Indices=1  OutputSizes=1
  Data Store Write3 : DataStoreWrite  DataStoreName=Start_STOP_TIMER_up  IndexOptions=Index vector (dialog)  Indices=1  OutputSizes=1
  Data Type Conversion : DataTypeConversion  Commented=on  OutDataTypeStr=double
  PWM Generator (DC-DC)1 : spsPWMGeneratorDCDCLib/PWM Generator (DC-DC)  Fsw=65e3  Ts=0
  Subtract : Sum  Inputs=-+
  Subtract1 : Sum  Inputs=+-
  Switch : Switch  Criteria=u2 > Threshold
  Switch1 : Switch  Commented=on  Criteria=u2 > Threshold
  Outport : Outport
  Outport1 : Outport  Port=2
  Outport2 : Outport  Port=3
  Outport3 : Outport  Port=4
  wires:
  Constant1/1 -> Switch/3
  Constant2/1 -> Subtract/2
  Constant/1 -> Switch/1
  AC/ input/1 -> Compare To Zero/1, Compare To Constant/1, Switch/2
  Switch/1 -> Outport1/1, Subtract/1
  Subtract/1 -> Outport/1
  Constant5/1 -> Data Store Write1/1
  Constant3/1 -> Subtract1/1
  Subtract1/1 -> Outport3/1
  PWM Generator (DC-DC)1/1 -> Subtract1/2, Outport2/1
  Compare To Constant/1 -> AND/1
  Compare To Zero/1 -> AND/2
  AND/1 -> Data Type Conversion/1
  Data Type Conversion/1 -> Switch1/2
  Constant6/1 -> Switch1/1
  Constant7/1 -> Switch1/3
  Switch1/1 -> ?
  PID output/1 -> PWM Generator (DC-DC)1/1
  Constant4/1 -> Data Store Write3/1

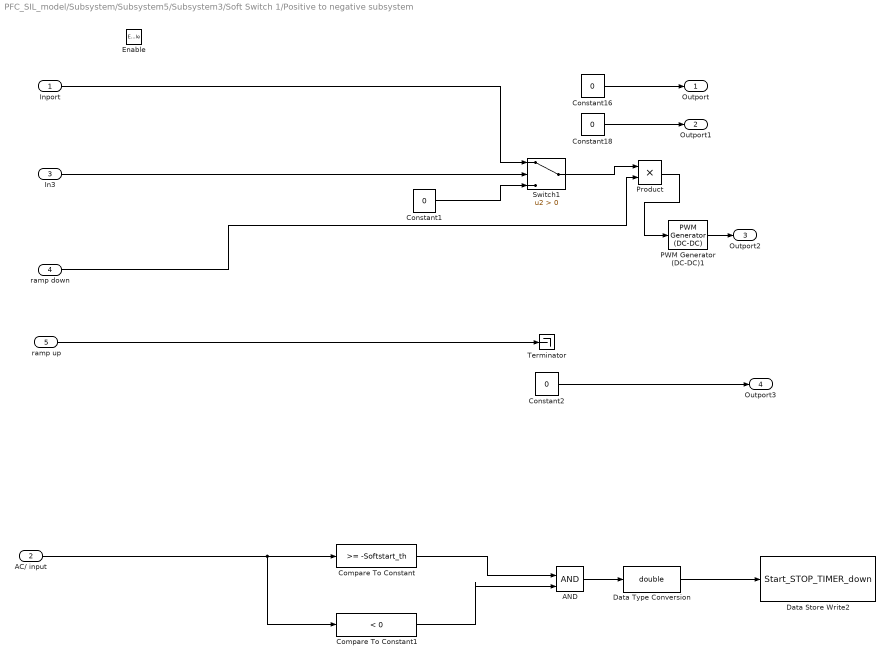
== system PFC_SIL_model/Subsystem/Subsystem5/Subsystem3/Soft Switch 1/Positive to negative subsystem  ==
  Inport : Inport
  AC/ input : Inport  Port=2
  In3 : Inport  Port=3
  "ramp down " : Inport  Port=4
  ramp up : Inport  Port=5
  Enable : EnablePort
  AND : Logic  IconShape=distinctive  AllPortsSameDT=off  OutDataTypeStr=boolean
  Compare To Constant : simulink/Logic and Bit Operations/Compare To Constant  relop=>=  const=-Softstart_th  OutDataTypeStr=boolean
  Compare To Constant1 : simulink/Logic and Bit Operations/Compare To Constant  relop=<  const=0  OutDataTypeStr=boolean
  Constant{1..2,16,18} (4 alike) : Constant  Value=0
  Data Store Write2 : DataStoreWrite  DataStoreName=Start_STOP_TIMER_down  IndexOptions=Index vector (dialog)  Indices=1  OutputSizes=1
  Data Type Conversion : DataTypeConversion  OutDataTypeStr=double
  PWM Generator (DC-DC)1 : spsPWMGeneratorDCDCLib/PWM Generator (DC-DC)  Fsw=65e3  Ts=0
  Product : Product
  Switch1 : Switch  Criteria=u2 > Threshold
  Terminator : Terminator
  Outport : Outport
  Outport1 : Outport  Port=2
  Outport2 : Outport  Port=3
  Outport3 : Outport  Port=4
  wires:
  Constant18/1 -> Outport1/1
  Constant16/1 -> Outport/1
  Inport/1 -> Switch1/1
  Compare To Constant/1 -> AND/1
  Compare To Constant1/1 -> AND/2
  AND/1 -> Data Type Conversion/1
  Data Type Conversion/1 -> Data Store Write2/1
  Switch1/1 -> Product/1
  Constant1/1 -> Switch1/3
  In3/1 -> Switch1/2
  Product/1 -> PWM Generator (DC-DC)1/1
  "ramp down "/1 -> Product/2
  Constant2/1 -> Outport3/1
  AC/ input/1 -> Compare To Constant/1, Compare To Constant1/1
  ramp up/1 -> Terminator/1
  PWM Generator (DC-DC)1/1 -> Outport2/1

== system PFC_SIL_model/Subsystem/Subsystem5/Subsystem3/Soft Switch 1/Ramp up  ==
  Enable : Inport
  Constant1 : Constant  Value=Ramp
  Ramp Generator : Subsystem
  Saturation : Saturate  UpperLimit=ramp_sat_max  LowerLimit=ramp_sat_min
  Outport : Outport
  wires:
  Saturation/1 -> Outport/1
  Ramp Generator/1(Ramp) -> Saturation/1
  Constant1/1 -> Ramp Generator/1(Ramp_Time)
  Enable/1 -> Ramp Generator/2(Enable)

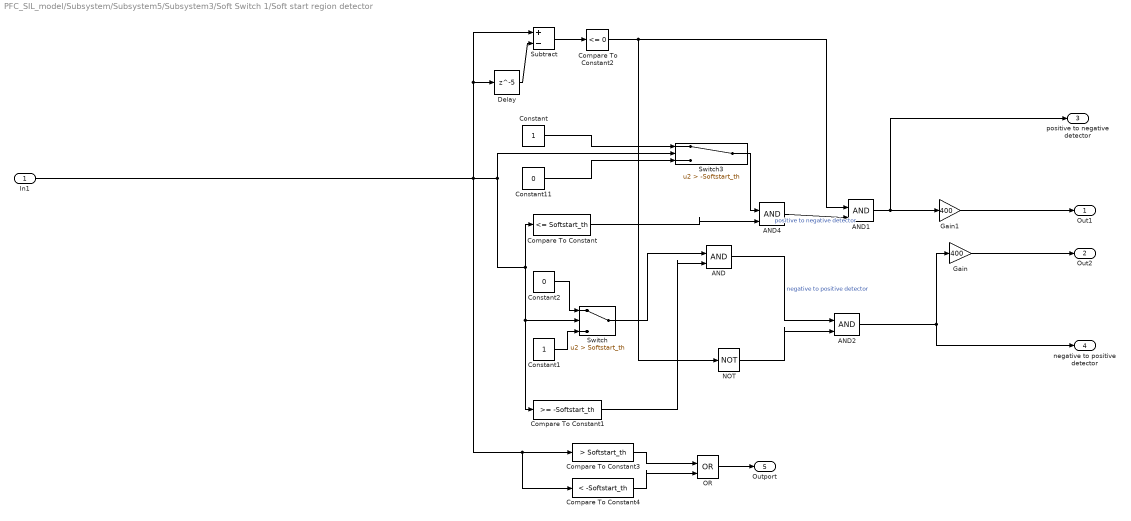
== system PFC_SIL_model/Subsystem/Subsystem5/Subsystem3/Soft Switch 1/Soft start region detector  ==
  In1 : Inport
  AND{,1..2,4} (4 alike) : Logic  IconShape=distinctive  AllPortsSameDT=off  OutDataTypeStr=boolean
  Compare To Constant : simulink/Logic and Bit Operations/Compare To Constant  relop=<=  const=Softstart_th  OutDataTypeStr=boolean
  Compare To Constant1 : simulink/Logic and Bit Operations/Compare To Constant  relop=>=  const=-Softstart_th  OutDataTypeStr=boolean
  Compare To Constant2 : simulink/Logic and Bit Operations/Compare To Constant  relop=<=  const=0  OutDataTypeStr=boolean
  Compare To Constant3 : simulink/Logic and Bit Operations/Compare To Constant  relop=>  const=Softstart_th  OutDataTypeStr=boolean
  Compare To Constant4 : simulink/Logic and Bit Operations/Compare To Constant  relop=<  const=-Softstart_th  OutDataTypeStr=boolean
  Constant : Constant
  Constant1 : Constant
  Constant11 : Constant  Value=0
  Constant2 : Constant  Value=0
  Delay : Delay  DelayLength=5
  Gain : Gain  Gain=400
  Gain1 : Gain  Gain=400
  NOT : Logic  Operator=NOT  IconShape=distinctive  AllPortsSameDT=off  OutDataTypeStr=boolean
  OR : Logic  Operator=OR  IconShape=distinctive  AllPortsSameDT=off  OutDataTypeStr=boolean
  Subtract : Sum  Inputs=+-
  Switch : Switch  Criteria=u2 > Threshold  Threshold=Softstart_th
  Switch3 : Switch  Criteria=u2 > Threshold  Threshold=-Softstart_th
  Out1 : Outport
  Out2 : Outport  Port=2
  positive to negative detector : Outport  Port=3
  negative to positive detector : Outport  Port=4
  Outport : Outport  Port=5
  wires:
  AND4/1 -> AND1/2  "positive to negative detector"
  Constant11/1 -> Switch3/3
  In1/1 -> Compare To Constant4/1, Compare To Constant3/1, Delay/1, Subtract/1, Switch3/2, Compare To Constant1/1, Switch/2, Compare To Constant/1
  Compare To Constant/1 -> AND4/2
  AND/1 -> AND2/1  "negative to positive detector"
  Switch3/1 -> AND4/1
  Constant/1 -> Switch3/1
  Gain1/1 -> Out1/1
  Gain/1 -> Out2/1
  Constant1/1 -> Switch/3
  Constant2/1 -> Switch/1
  Switch/1 -> AND/1
  Compare To Constant1/1 -> AND/2
  Delay/1 -> Subtract/2
  Subtract/1 -> Compare To Constant2/1
  Compare To Constant2/1 -> NOT/1, AND1/1
  NOT/1 -> AND2/2
  AND2/1 -> Gain/1, negative to positive detector/1
  AND1/1 -> positive to negative detector/1, Gain1/1
  Compare To Constant3/1 -> OR/1
  Compare To Constant4/1 -> OR/2
  OR/1 -> Outport/1

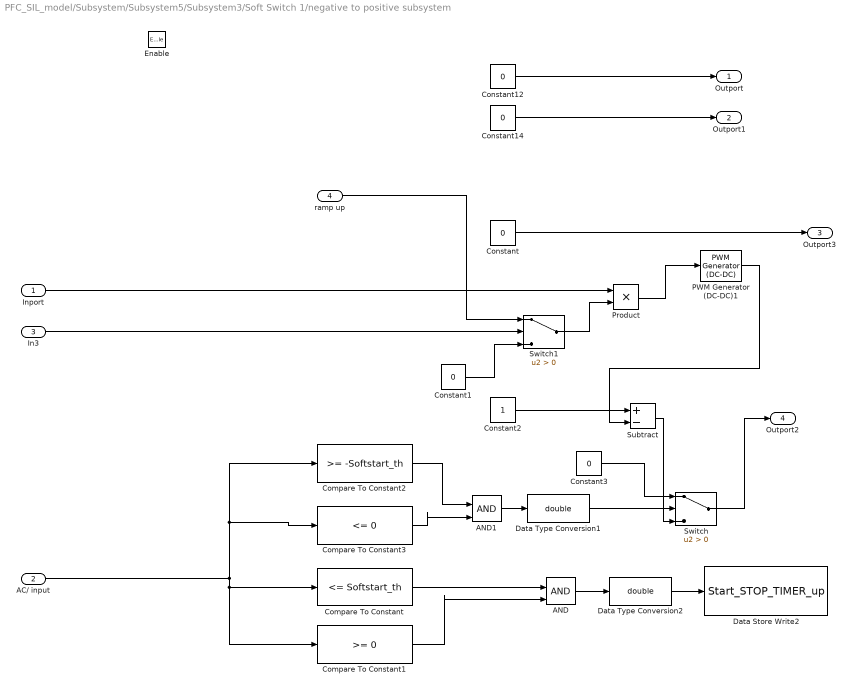
== system PFC_SIL_model/Subsystem/Subsystem5/Subsystem3/Soft Switch 1/negative to positive subsystem  ==
  Inport : Inport
  AC/ input : Inport  Port=2
  In3 : Inport  Port=3
  "ramp up " : Inport  Port=4
  Enable : EnablePort
  AND : Logic  IconShape=distinctive  AllPortsSameDT=off  OutDataTypeStr=boolean
  AND1 : Logic  IconShape=distinctive  AllPortsSameDT=off  OutDataTypeStr=boolean
  Compare To Constant : simulink/Logic and Bit Operations/Compare To Constant  relop=<=  const=Softstart_th  OutDataTypeStr=boolean
  Compare To Constant1 : simulink/Logic and Bit Operations/Compare To Constant  relop=>=  const=0  OutDataTypeStr=boolean
  Compare To Constant2 : simulink/Logic and Bit Operations/Compare To Constant  relop=>=  const=-Softstart_th  OutDataTypeStr=boolean
  Compare To Constant3 : simulink/Logic and Bit Operations/Compare To Constant  relop=<=  const=0  OutDataTypeStr=boolean
  Constant{,1,3,12,14} (5 alike) : Constant  Value=0
  Constant2 : Constant
  Data Store Write2 : DataStoreWrite  DataStoreName=Start_STOP_TIMER_up  IndexOptions=Index vector (dialog)  Indices=1  OutputSizes=1
  Data Type Conversion1 : DataTypeConversion  OutDataTypeStr=double
  Data Type Conversion2 : DataTypeConversion  OutDataTypeStr=double
  PWM Generator (DC-DC)1 : spsPWMGeneratorDCDCLib/PWM Generator (DC-DC)  Fsw=65e3  Ts=0
  Product : Product
  Subtract : Sum  Inputs=+-
  Switch : Switch  Criteria=u2 > Threshold
  Switch1 : Switch  Criteria=u2 > Threshold
  Outport : Outport
  Outport1 : Outport  Port=2
  Outport3 : Outport  Port=3
  Outport2 : Outport  Port=4
  wires:
  Constant12/1 -> Outport/1
  Constant14/1 -> Outport1/1
  AC/ input/1 -> Compare To Constant3/1, Compare To Constant2/1, Compare To Constant/1, Compare To Constant1/1
  Compare To Constant/1 -> AND/1
  Compare To Constant1/1 -> AND/2
  AND/1 -> Data Type Conversion2/1
  Data Type Conversion2/1 -> Data Store Write2/1
  Constant1/1 -> Switch1/3
  Switch1/1 -> Product/2
  In3/1 -> Switch1/2
  Inport/1 -> Product/1
  "ramp up "/1 -> Switch1/1
  Product/1 -> PWM Generator (DC-DC)1/1
  Constant/1 -> Outport3/1
  PWM Generator (DC-DC)1/1 -> Subtract/2
  Constant2/1 -> Subtract/1
  Subtract/1 -> Switch/3
  Compare To Constant2/1 -> AND1/1
  Compare To Constant3/1 -> AND1/2
  AND1/1 -> Data Type Conversion1/1
  Data Type Conversion1/1 -> Switch/2
  Constant3/1 -> Switch/1
  Switch/1 -> Outport2/1

== system PFC_SIL_model/Subsystem/Subsystem5/Subsystem3/Soft Switch 1/ramp down ==
  Enable : Inport
  Constant : Constant
  Constant1 : Constant  Value=Ramp
  Ramp Generator : Subsystem
  Saturation : Saturate  UpperLimit=ramp_sat_max  LowerLimit=ramp_sat_min
  Subtract : Sum  Inputs=+-
  Outport : Outport
  wires:
  Saturation/1 -> Subtract/2
  Ramp Generator/1(Ramp) -> Saturation/1
  Constant1/1 -> Ramp Generator/1(Ramp_Time)
  Enable/1 -> Ramp Generator/2(Enable)
  Constant/1 -> Subtract/1
  Subtract/1 -> Outport/1
